simulink model "CardioVascularSystemWithEcmo"  (R2021b)
settings: Solver=daessc  StartTime=0.0  StopTime=Tend  MaxStep=0.6  RelTol=1e-3  AbsTol=1e-3
undefined symbols (not defined in the file): EsL, EsR, PipL, PipR, R1, R2, R3, R4, R5, R6, R7, R8, RL, RPM_Setting, RR, SetHartRate, tc, ts, WaitTime
libraries: fl_lib x66, nesl_utility x24, ee_lib x4, SignalEditorBlockLib x1
settings Model: Creator=mnord  LastModifiedBy=mnord
settings SolverCC: ZeroCrossAlgorithm=Adaptive  AlgebraicLoopSolver=TrustRegion
settings DebuggingCC: MaxConsecutiveZCsMsg=warning  IgnoredZcDiagnostic=none  SymbolicDimsDataTypeCodeGenerationDiagnostic=none  SFMachineParentedDataDiag=warning
settings SFSimCC: CustomCodeUndefinedFunction=UseInterfaceOnly
settings SimscapeCC: SimscapeLogType=all  SimscapeLogSimulationStatistics=on  SimscapeLogDataHistory=10000

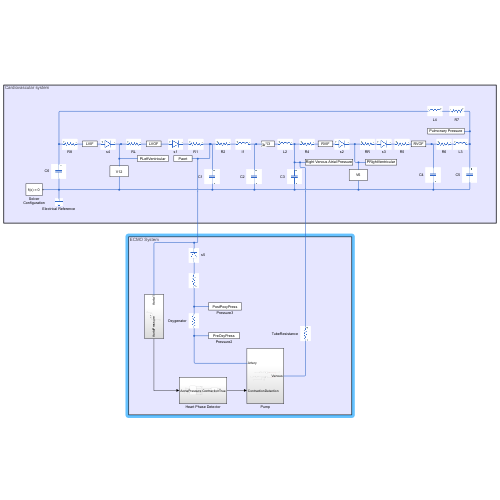
[thumbnail: Simulink's stored preview of the top-level diagram]
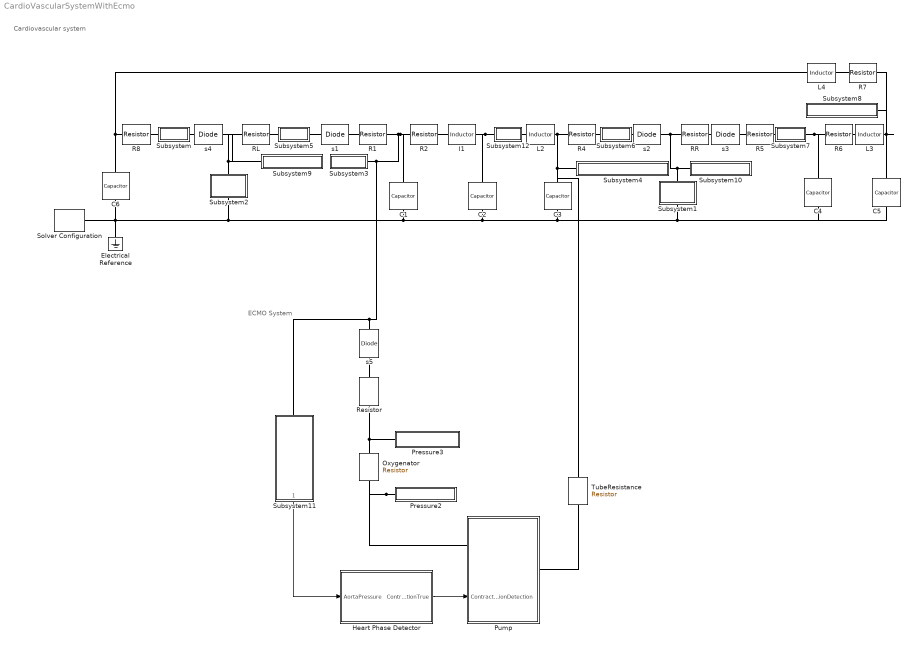
== system CardioVascularSystemWithEcmo ==
  note: Cardiovascular system
  note: ECMO System
  C1 : fl_lib/Electrical/Electrical Elements/Capacitor  c=C1 F  r=capSerRes Ohm  g=0 1/Ohm  i_specify=off  i_priority=None  i=0 A  i_nominal_specify=off  i_nominal_unit=A  i_nominal_value=1  v_specify=off  v_priority=High  v=X10 V  v_nominal_specify=off  v_nominal_unit=V  v_nominal_value=1  vc_specify=on  vc_priority=High  vc=X10 V  vc_nominal_specify=off  vc_nominal_unit=V  vc_nominal_value=1
  C2 : fl_lib/Electrical/Electrical Elements/Capacitor  c=C2 F  r=capSerRes Ohm  g=0 1/Ohm  i_specify=off  i_priority=None  i=0 A  i_nominal_specify=off  i_nominal_unit=A  i_nominal_value=1  v_specify=off  v_priority=High  v=X30 V  v_nominal_specify=off  v_nominal_unit=V  v_nominal_value=1  vc_specify=on  vc_priority=High  vc=X30 V  vc_nominal_specify=off  vc_nominal_unit=V  vc_nominal_value=1
  C3 : fl_lib/Electrical/Electrical Elements/Capacitor  c=C3 F  r=capSerRes Ohm  g=0 1/Ohm  i_specify=off  i_priority=None  i=0 A  i_nominal_specify=off  i_nominal_unit=A  i_nominal_value=1  v_specify=off  v_priority=High  v=X50 V  v_nominal_specify=off  v_nominal_unit=V  v_nominal_value=1  vc_specify=on  vc_priority=High  vc=X50 V  vc_nominal_specify=off  vc_nominal_unit=V  vc_nominal_value=1
  C4 : fl_lib/Electrical/Electrical Elements/Capacitor  c=C4 F  r=capSerRes Ohm  g=0 1/Ohm  i_specify=off  i_priority=None  i=0 A  i_nominal_specify=off  i_nominal_unit=A  i_nominal_value=1  v_specify=off  v_priority=High  v=X70 V  v_nominal_specify=off  v_nominal_unit=V  v_nominal_value=1  vc_specify=on  vc_priority=High  vc=X70 V  vc_nominal_specify=off  vc_nominal_unit=V  vc_nominal_value=1
  C5 : fl_lib/Electrical/Electrical Elements/Capacitor  c=C5 F  r=capSerRes Ohm  g=0 1/Ohm  i_specify=off  i_priority=None  i=0 A  i_nominal_specify=off  i_nominal_unit=A  i_nominal_value=1  v_specify=off  v_priority=High  v=X90 V  v_nominal_specify=off  v_nominal_unit=V  v_nominal_value=1  vc_specify=on  vc_priority=High  vc=X90 V  vc_nominal_specify=off  vc_nominal_unit=V  vc_nominal_value=1
  C6 : fl_lib/Electrical/Electrical Elements/Capacitor  c=C6 F  r=capSerRes Ohm  g=0 1/Ohm  i_specify=off  i_priority=None  i=0 A  i_nominal_specify=off  i_nominal_unit=A  i_nominal_value=1  v_specify=off  v_priority=High  v=X110 V  v_nominal_specify=off  v_nominal_unit=V  v_nominal_value=1  vc_specify=on  vc_priority=High  vc=X110 V  vc_nominal_specify=off  vc_nominal_unit=V  vc_nominal_value=1
  Electrical Reference : fl_lib/Electrical/Electrical Elements/Electrical Reference
  Heart Phase Detector : Subsystem
  I1 : ee_lib/Passive/Inductor  l=L1 H  L_tol=20  enable_L_tol=0  tol_distribution=1  nSigma=4  r=0 Ohm  g=1e-9 1/Ohm  enable_operating_limits=0  operating_limit_action=2  max_working_current=1 A  power_rating=1 W  enable_faults=0  fault_action=1  lambdaPercent=50  k_faulted=0.9999  turnsShort=0  openCct=0  groundShort=0  groundShortG=0 1/Ohm  tau_fault=1e-3 s  enable_temporal_fault=0  t_fault=1 s  enable_behavioral_fault=0  max_permissible_voltage=100 V  n_fail_on_voltage=1  max_permissible_current=1 A  t_fail_on_current=1 s  i_L_specify=on  i_L_priority=High  i_L=X20 A  i_L_nominal_specify=off  i_L_nominal_unit=A  i_L_nominal_value=1
  L2 : ee_lib/Passive/Inductor  l=L2 H  L_tol=20  enable_L_tol=0  tol_distribution=1  nSigma=4  r=0 Ohm  g=1e-9 1/Ohm  enable_operating_limits=0  operating_limit_action=2  max_working_current=1 A  power_rating=1 W  enable_faults=0  fault_action=1  lambdaPercent=50  k_faulted=0.9999  turnsShort=0  openCct=0  groundShort=0  groundShortG=0 1/Ohm  tau_fault=1e-3 s  enable_temporal_fault=0  t_fault=1 s  enable_behavioral_fault=0  max_permissible_voltage=100 V  n_fail_on_voltage=1  max_permissible_current=1 A  t_fail_on_current=1 s  i_L_specify=on  i_L_priority=High  i_L=X40 A  i_L_nominal_specify=off  i_L_nominal_unit=A  i_L_nominal_value=1
  L3 : ee_lib/Passive/Inductor  l=L3 H  L_tol=20  enable_L_tol=0  tol_distribution=1  nSigma=4  r=0 Ohm  g=1e-9 1/Ohm  enable_operating_limits=0  operating_limit_action=2  max_working_current=1 A  power_rating=1 W  enable_faults=0  fault_action=1  lambdaPercent=50  k_faulted=0.9999  turnsShort=0  openCct=0  groundShort=0  groundShortG=0 1/Ohm  tau_fault=1e-3 s  enable_temporal_fault=0  t_fault=1 s  enable_behavioral_fault=0  max_permissible_voltage=100 V  n_fail_on_voltage=1  max_permissible_current=1 A  t_fail_on_current=1 s  i_L_specify=on  i_L_priority=High  i_L=X80 A  i_L_nominal_specify=off  i_L_nominal_unit=A  i_L_nominal_value=1
  L4 : ee_lib/Passive/Inductor  l=L4 H  L_tol=20  enable_L_tol=0  tol_distribution=1  nSigma=4  r=0 Ohm  g=1e-9 1/Ohm  enable_operating_limits=0  operating_limit_action=2  max_working_current=1 A  power_rating=1 W  enable_faults=0  fault_action=1  lambdaPercent=50  k_faulted=0.9999  turnsShort=0  openCct=0  groundShort=0  groundShortG=0 1/Ohm  tau_fault=1e-3 s  enable_temporal_fault=0  t_fault=1 s  enable_behavioral_fault=0  max_permissible_voltage=100 V  n_fail_on_voltage=1  max_permissible_current=1 A  t_fail_on_current=1 s  i_L_specify=on  i_L_priority=High  i_L=X100 A  i_L_nominal_specify=off  i_L_nominal_unit=A  i_L_nominal_value=1
  Oxygenator : fl_lib/Electrical/Electrical Elements/Resistor  R=1/1.13 Ohm  i_specify=off  i_priority=None  i=0 A  i_nominal_specify=off  i_nominal_unit=A  i_nominal_value=1  v_specify=off  v_priority=None  v=0 V  v_nominal_specify=off  v_nominal_unit=V  v_nominal_value=1
  Pressure2 : Subsystem
      mask Display: disp('PreOxyPress')
  Pressure3 : Subsystem
      mask Display: disp('PostPoxyPress')
  Pump : Subsystem
      settings: PortSchema="{\"entries\":[{\"content\":{\"sides\":[{\"content\":{\"connectorIds\":[\"LConn1\"]},\"type\":\"ConnectorPlacement.EquallySpacedRectSide\",\"uuid\":\"62db16dc-542a-4803-9c2c-9a470fc91885\"},{\"content\":{\"connectorIds\":[\"RConn1\",\"In1\"],\"side\":\"RIGHT\"},\"type\":\"ConnectorPlacement.EquallySpacedRectSide\",\"uuid\":\"05a4665e-1cd6-4c93-95ba-f78495d840a1\"},{\"content\":{\"connectorIds\":[],\"side\":\"TOP\"},\"type\":\"ConnectorPlacement.EquallySpacedRectSide\",\"uuid\":\"174192fa-e994-4b45-8a1f-dd44ebe2b866\"},{\"content\":{\"connectorIds\":[],\"side\":\"BOTTOM\"},\"type\":\"ConnectorPlacement.EquallySpacedRectSide\",\"uuid\":\"194a326f-2a13-4189-b0b8-d4f935dc1fe6\"}]},\"type\":\"ConnectorPlacement.EquallySpacedConnector\",\"uuid\":\"9d7b36c7-1763-48ea-a53e-009c812e3b66\"}],\"packageUris\":[\"http://schema.mathworks.com/mf0/Connector/R2020b\"],\"version\":\"1.0\"}"
  R1 : fl_lib/Electrical/Electrical Elements/Resistor  R=R1 Ohm  i_specify=off  i_priority=None  i=0 A  i_nominal_specify=off  i_nominal_unit=A  i_nominal_value=1  v_specify=off  v_priority=None  v=0 V  v_nominal_specify=off  v_nominal_unit=V  v_nominal_value=1
  R2 : fl_lib/Electrical/Electrical Elements/Resistor  R=R2 Ohm  i_specify=off  i_priority=None  i=0 A  i_nominal_specify=off  i_nominal_unit=A  i_nominal_value=1  v_specify=off  v_priority=None  v=0 V  v_nominal_specify=off  v_nominal_unit=V  v_nominal_value=1
  R4 : fl_lib/Electrical/Electrical Elements/Resistor  R=R4 Ohm  i_specify=off  i_priority=None  i=0 A  i_nominal_specify=off  i_nominal_unit=A  i_nominal_value=1  v_specify=off  v_priority=None  v=0 V  v_nominal_specify=off  v_nominal_unit=V  v_nominal_value=1
  R5 : fl_lib/Electrical/Electrical Elements/Resistor  R=R5 Ohm  i_specify=off  i_priority=None  i=0 A  i_nominal_specify=off  i_nominal_unit=A  i_nominal_value=1  v_specify=off  v_priority=None  v=0 V  v_nominal_specify=off  v_nominal_unit=V  v_nominal_value=1
  R6 : fl_lib/Electrical/Electrical Elements/Resistor  R=R6 Ohm  i_specify=off  i_priority=None  i=0 A  i_nominal_specify=off  i_nominal_unit=A  i_nominal_value=1  v_specify=off  v_priority=None  v=0 V  v_nominal_specify=off  v_nominal_unit=V  v_nominal_value=1
  R7 : fl_lib/Electrical/Electrical Elements/Resistor  R=R7 Ohm  i_specify=off  i_priority=None  i=0 A  i_nominal_specify=off  i_nominal_unit=A  i_nominal_value=1  v_specify=off  v_priority=None  v=0 V  v_nominal_specify=off  v_nominal_unit=V  v_nominal_value=1
  R8 : fl_lib/Electrical/Electrical Elements/Resistor  R=R8 Ohm  i_specify=off  i_priority=None  i=0 A  i_nominal_specify=off  i_nominal_unit=A  i_nominal_value=1  v_specify=off  v_priority=None  v=0 V  v_nominal_specify=off  v_nominal_unit=V  v_nominal_value=1
  RL : fl_lib/Electrical/Electrical Elements/Resistor  R=RL Ohm  i_specify=off  i_priority=None  i=0 A  i_nominal_specify=off  i_nominal_unit=A  i_nominal_value=1  v_specify=off  v_priority=None  v=0 V  v_nominal_specify=off  v_nominal_unit=V  v_nominal_value=1
  RR : fl_lib/Electrical/Electrical Elements/Resistor  R=RR Ohm  i_specify=off  i_priority=None  i=0 A  i_nominal_specify=off  i_nominal_unit=A  i_nominal_value=1  v_specify=off  v_priority=None  v=0 V  v_nominal_specify=off  v_nominal_unit=V  v_nominal_value=1
  Resistor : fl_lib/Electrical/Electrical Elements/Resistor  R=1/1.6 Ohm  i_specify=off  i_priority=None  i=0 A  i_nominal_specify=off  i_nominal_unit=A  i_nominal_value=1  v_specify=off  v_priority=None  v=0 V  v_nominal_specify=off  v_nominal_unit=V  v_nominal_value=1
  Solver Configuration : nesl_utility/Solver Configuration  PhysicalDomain=network_engine_domain  SubClassName=solver  LeftPortType=input  RightPortType=generic  Tones=[]  Harmonics=[]  SimulateNoise=off  Profile=off  UseLocalSampling=off  EnableSwitchedLinearOptims=on  FrequencyDomain=off  UseCCode=off  RelTol=0.001  AbsTol=1e-06  MinStep=1e-09  ToWorkspace=off  RevertToSquareIcSolve=off  NumHomotopyIterations=100  PhasorMode=off  PhasorModeNumHarmonics=1  DoDC=off  ResidualTolerance=1e-09  UseLocalSolver=off  LocalSolverChoice=NE_BACKWARD_EULER_ADVANCER  LocalSolverSampleTime=0.001  DoFixedCost=off  MaxNonlinIter=3  MaxModeIter=2  ComputeImpulses=off  ImpulseIterations=2  LinearAlgebra=auto  EquationFormulation=NE_TIME_EF  DelaysMemoryBudget=1024  AutomaticFiltering=on  FilteringTimeConstant=0.001  PartitionStorageMethod=AS_NEEDED  PartitionMemoryBudget=1024  PartitionMethod=ROBUST
      settings: SourceProductBaseCode=PW,SS
  Subsystem : Subsystem
      mask Display: disp('LVIF')
  Subsystem1 : Subsystem
      mask Display: disp('V6')
  Subsystem10 : Subsystem
      mask Display: disp('PRightVentricular')
  Subsystem11 : Subsystem
      settings: PortSchema="{\"entries\":[{\"content\":{\"sides\":[{\"content\":{\"connectorIds\":[]},\"type\":\"ConnectorPlacement.EquallySpacedRectSide\",\"uuid\":\"f9ffc3b3-0f3f-4df5-be7e-a65199d8fb18\"},{\"content\":{\"connectorIds\":[],\"side\":\"RIGHT\"},\"type\":\"ConnectorPlacement.EquallySpacedRectSide\",\"uuid\":\"6b3c46a3-b656-482e-b0a9-93777308e083\"},{\"content\":{\"connectorIds\":[\"LConn1\"],\"side\":\"TOP\"},\"type\":\"ConnectorPlacement.EquallySpacedRectSide\",\"uuid\":\"e2309b6a-a528-4e82-8df5-2fdb2444f40a\"},{\"content\":{\"connectorIds\":[\"Out1\"],\"side\":\"BOTTOM\"},\"type\":\"ConnectorPlacement.EquallySpacedRectSide\",\"uuid\":\"7e89f23f-224f-485d-9e96-fb39bd2403a7\"}]},\"type\":\"ConnectorPlacement.EquallySpacedConnector\",\"uuid\":\"798f20cf-0f77-4082-bc02-f5f2bf5391c0\"}],\"packageUris\":[\"http://schema.mathworks.com/mf0/Connector/R2020b\"],\"version\":\"1.0\"}"
  Subsystem12 : Subsystem  Variant=on  VariantControlMode=label  VariantControl=Choice  LabelModeActiveChoice=R3_Fix
      mask Display: disp('R3')
  Subsystem2 : Subsystem
      mask Display: disp('V12')
  Subsystem3 : Subsystem
      mask Display: disp('Paort')
  Subsystem4 : Subsystem
      mask Display: disp('Right Venous Atrial Pressure')
  Subsystem5 : Subsystem
      mask Display: disp('LVOF')
  Subsystem6 : Subsystem
      mask Display: disp('RVIF')
  Subsystem7 : Subsystem
      mask Display: disp('RVOF')
  Subsystem8 : Subsystem
      mask Display: disp('Pulmonary Pressure')
  Subsystem9 : Subsystem
      mask Display: disp('PLeftVentricular')
  TubeResistance : fl_lib/Electrical/Electrical Elements/Resistor  R=1 Ohm  i_specify=off  i_priority=None  i=60 A  i_nominal_specify=off  i_nominal_unit=A  i_nominal_value=1  v_specify=off  v_priority=None  v=0 V  v_nominal_specify=off  v_nominal_unit=V  v_nominal_value=1
  s{1..4} (4 alike) : fl_lib/Electrical/Electrical Elements/Diode  Vf=FwVolt V  Ron=onRes Ohm  Goff=1e-8 1/Ohm  i_specify=off  i_priority=None  i=0 A  i_nominal_specify=off  i_nominal_unit=A  i_nominal_value=1  v_specify=off  v_priority=None  v=0 V  v_nominal_specify=off  v_nominal_unit=V  v_nominal_value=1
  s5 : fl_lib/Electrical/Electrical Elements/Diode  Vf=FwVolt V  Ron=0.54*0.1 Ohm  Goff=1e-8 1/Ohm  i_specify=off  i_priority=None  i=0 A  i_nominal_specify=off  i_nominal_unit=A  i_nominal_value=1  v_specify=off  v_priority=None  v=0 V  v_nominal_specify=off  v_nominal_unit=V  v_nominal_value=1
  wires:
  Subsystem11/1(AortaPressure) -> Heart Phase Detector/1(AortaPressure)
  Heart Phase Detector/1(ContractionTrue) -> Pump/1(ContractionDetection)
  connections:
  R2/RConn1 -- I1/LConn1
  s1/LConn1 -- Subsystem5/RConn1
  s2/LConn1 -- Subsystem6/RConn1
  R5/RConn1 -- Subsystem7/LConn1
  s4/LConn1 -- Subsystem/RConn1
  R6/LConn1 -- C4/LConn1 -- Subsystem7/RConn1
  Subsystem12/RConn1 -- L2/LConn1
  Subsystem5/LConn1 -- RL/RConn1
  L3/RConn1 -- Subsystem8/LConn1 -- R7/LConn1 -- C5/LConn1
  Subsystem6/LConn1 -- R4/RConn1
  C6/LConn1 -- R8/LConn1 -- L4/RConn1
  s1/RConn1 -- R1/LConn1
  s3/RConn1 -- R5/LConn1
  L3/LConn1 -- R6/RConn1
  R7/RConn1 -- L4/LConn1
  R8/RConn1 -- Subsystem/LConn1
  Subsystem10/LConn1 -- Subsystem1/LConn1 -- RR/LConn1 -- s2/RConn1
  s4/RConn1 -- RL/LConn1 -- Subsystem9/LConn1 -- Subsystem2/LConn1
  s3/LConn1 -- RR/RConn1
  C6/RConn1 -- Electrical Reference/LConn1 -- C5/RConn1 -- C4/RConn1 -- Subsystem1/RConn1 -- C3/RConn1 -- C2/RConn1 -- C1/RConn1 -- Subsystem2/RConn1 -- Solver Configuration/RConn1
  I1/RConn1 -- C2/LConn1 -- Subsystem12/LConn1
  Pressure2/RConn1 -- Pump/RConn1 -- Oxygenator/LConn1
  R4/LConn1 -- TubeResistance/LConn1 -- Subsystem4/LConn1 -- C3/LConn1 -- L2/RConn1
  Resistor/RConn1 -- s5/LConn1
  Oxygenator/RConn1 -- Resistor/LConn1 -- Pressure3/RConn1
  Pump/LConn1 -- TubeResistance/RConn1
  C1/LConn1 -- R1/RConn1 -- Subsystem11/LConn1 -- s5/RConn1 -- Subsystem3/LConn1 -- R2/LConn1

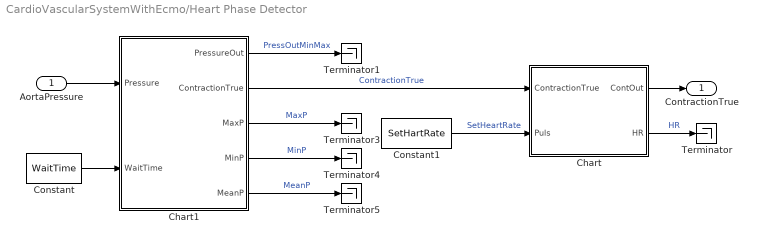
== system CardioVascularSystemWithEcmo/Heart Phase Detector ==
  AortaPressure : Inport
  Chart : Stateflow chart  TreatAsAtomicUnit=on
  Chart1 : Stateflow chart  TreatAsAtomicUnit=on
  Constant : Constant  Value=WaitTime
  Constant1 : Constant  Value=SetHartRate
  Terminator{,1,3..5} (5 alike) : Terminator
  ContractionTrue : Outport
  wires:
  AortaPressure/1 -> Chart1/1(Pressure)
  Chart1/1(PressureOut) -> Terminator1/1  "PressOutMinMax"
  Chart1/2(ContractionTrue) -> Chart/1(ContractionTrue)  "ContractionTrue"
  Chart1/4(MinP) -> Terminator4/1  "MinP"
  Chart1/3(MaxP) -> Terminator3/1  "MaxP"
  Chart1/5(MeanP) -> Terminator5/1  "MeanP"
  Constant/1 -> Chart1/2(WaitTime)
  Chart/1(ContOut) -> ContractionTrue/1
  Chart/2(HR) -> Terminator/1  "HR"
  Constant1/1 -> Chart/2(Puls)  "SetHeartRate"

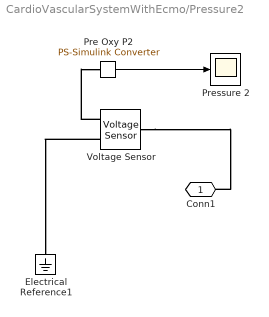
== system CardioVascularSystemWithEcmo/Pressure2 ==
  Electrical Reference1 : fl_lib/Electrical/Electrical Elements/Electrical Reference
  Pre Oxy P2 : nesl_utility/PS-Simulink Converter  PhysicalDomain=network_engine_domain  SubClassName=ps_output  LeftPortType=input  RightPortType=output  PseudoPeriodic=off  Frequencies=[]  Unit=inherit  AffineConversion=off
      settings: SourceProductBaseCode=PW,SS
  Pressure 2 : Scope
  Voltage Sensor : fl_lib/Electrical/Electrical Sensors/Voltage Sensor
  Conn1 : PMIOPort  Side=Right
  wires:
  Pre Oxy P2/1 -> Pressure 2/1
  connections:
  Voltage Sensor/RConn1 -- Pre Oxy P2/LConn1
  Voltage Sensor/LConn1 -- Conn1/RConn1
  Voltage Sensor/RConn2 -- Electrical Reference1/LConn1

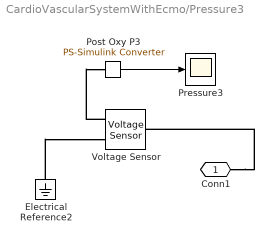
== system CardioVascularSystemWithEcmo/Pressure3 ==
  Electrical Reference2 : fl_lib/Electrical/Electrical Elements/Electrical Reference
  Post Oxy P3 : nesl_utility/PS-Simulink Converter  PhysicalDomain=network_engine_domain  SubClassName=ps_output  LeftPortType=input  RightPortType=output  PseudoPeriodic=off  Frequencies=[]  Unit=inherit  AffineConversion=off
      settings: SourceProductBaseCode=PW,SS
  Pressure3 : Scope
  Voltage Sensor : fl_lib/Electrical/Electrical Sensors/Voltage Sensor
  Conn1 : PMIOPort  Side=Right
  wires:
  Post Oxy P3/1 -> Pressure3/1
  connections:
  Voltage Sensor/RConn1 -- Post Oxy P3/LConn1
  Electrical Reference2/LConn1 -- Voltage Sensor/RConn2
  Conn1/RConn1 -- Voltage Sensor/LConn1

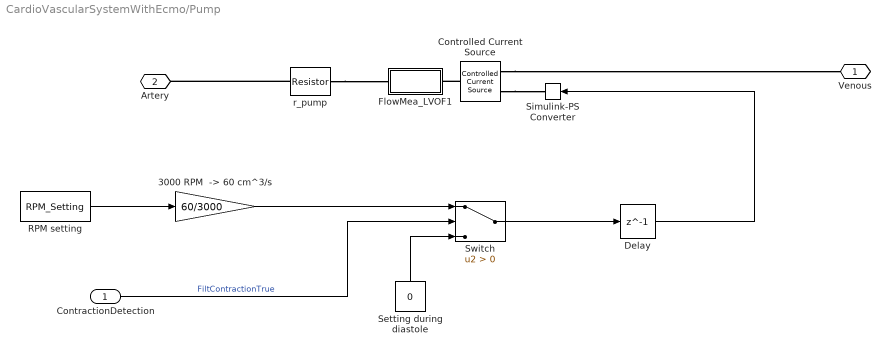
== system CardioVascularSystemWithEcmo/Pump ==
  ContractionDetection : Inport
  "3000 RPM  -> 60 cm^3/s" : Gain  Gain=60/3000
  Controlled Current Source : fl_lib/Electrical/Electrical Sources/Controlled Current Source
  Delay : Delay  DelayLength=1  SampleTime=0.001
  FlowMea_LVOF1 : Subsystem
      mask Display: disp('EcmoFlow')
  RPM setting : Constant  Value=RPM_Setting
  Setting during diastole : Constant  Value=0
  Simulink-PS Converter : nesl_utility/Simulink-PS Converter  PhysicalDomain=network_engine_domain  SubClassName=ps_input  LeftPortType=input  RightPortType=output  PseudoPeriodic=off  Frequencies=[]  NoiseDistribution=none  NoiseParameters=[]  Unit=1  AffineConversion=off  FilteringAndDerivatives=filter  SimscapeFilterOrder=1  InputFilterTimeConstant=0.001  UdotUserProvided=0
      settings: SourceProductBaseCode=PW,SS
  Switch : Switch  Criteria=u2 > Threshold
  r_pump : fl_lib/Electrical/Electrical Elements/Resistor  R=1/1.68 Ohm  i_specify=on  i_priority=None  i=83.3 A  i_nominal_specify=off  i_nominal_unit=A  i_nominal_value=1  v_specify=off  v_priority=None  v=0 V  v_nominal_specify=off  v_nominal_unit=V  v_nominal_value=1
  Venous : PMIOPort  Side=Left
  Artery : PMIOPort  Port=2  Side=Right
  wires:
  Delay/1 -> Simulink-PS Converter/1
  "3000 RPM  -> 60 cm^3/s"/1 -> Switch/1
  ContractionDetection/1 -> Switch/2  "FiltContractionTrue"
  RPM setting/1 -> "3000 RPM  -> 60 cm^3/s"/1
  Switch/1 -> Delay/1
  Setting during diastole/1 -> Switch/3
  connections:
  Controlled Current Source/RConn2 -- Venous/RConn1
  r_pump/LConn1 -- FlowMea_LVOF1/LConn1
  Controlled Current Source/RConn1 -- Simulink-PS Converter/RConn1
  r_pump/RConn1 -- Artery/RConn1
  Controlled Current Source/LConn1 -- FlowMea_LVOF1/RConn1

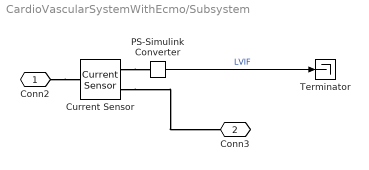
== system CardioVascularSystemWithEcmo/Subsystem ==
  Current Sensor : fl_lib/Electrical/Electrical Sensors/Current Sensor
  PS-Simulink Converter : nesl_utility/PS-Simulink Converter  PhysicalDomain=network_engine_domain  SubClassName=ps_output  LeftPortType=input  RightPortType=output  PseudoPeriodic=off  Frequencies=[]  Unit=inherit  AffineConversion=off
      settings: SourceProductBaseCode=PW,SS
  Terminator : Terminator
  Conn2 : PMIOPort  Side=Left
  Conn3 : PMIOPort  Port=2  Side=Right
  wires:
  PS-Simulink Converter/1 -> Terminator/1  "LVIF"
  connections:
  Conn2/RConn1 -- Current Sensor/LConn1
  Current Sensor/RConn2 -- Conn3/RConn1
  Current Sensor/RConn1 -- PS-Simulink Converter/LConn1

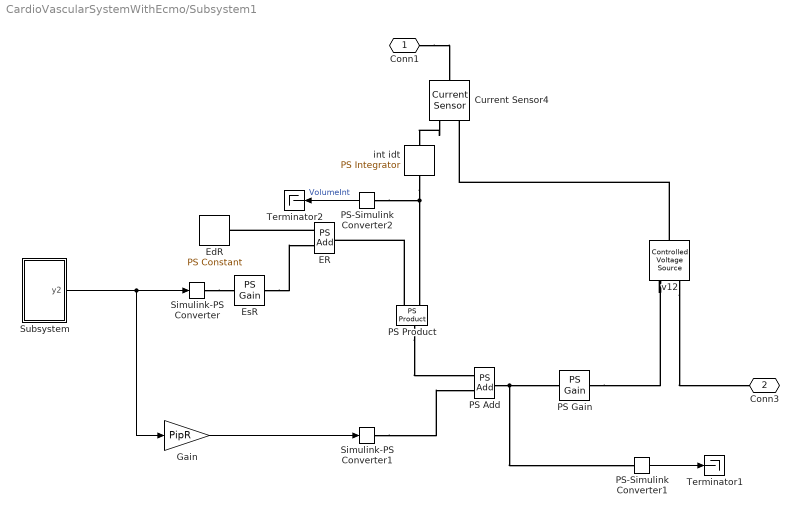
== system CardioVascularSystemWithEcmo/Subsystem1 ==
  Current Sensor4 : fl_lib/Electrical/Electrical Sensors/Current Sensor
  ER : fl_lib/Physical Signals/Functions/PS Add
  EdR : fl_lib/Physical Signals/Sources/PS Constant  constant=EdR
  EsR : fl_lib/Physical Signals/Functions/PS Gain  gain=EsR
  Gain : Gain  Gain=PipR
  PS Add : fl_lib/Physical Signals/Functions/PS Add
  PS Gain : fl_lib/Physical Signals/Functions/PS Gain  gain=1 V/s/A
  PS Product : fl_lib/Physical Signals/Functions/PS Product
  PS-Simulink Converter1 : nesl_utility/PS-Simulink Converter  PhysicalDomain=network_engine_domain  SubClassName=ps_output  LeftPortType=input  RightPortType=output  PseudoPeriodic=off  Frequencies=[]  Unit=inherit  AffineConversion=off
      settings: SourceProductBaseCode=PW,SS
  PS-Simulink Converter2 : nesl_utility/PS-Simulink Converter  PhysicalDomain=network_engine_domain  SubClassName=ps_output  LeftPortType=input  RightPortType=output  PseudoPeriodic=off  Frequencies=[]  Unit=inherit  AffineConversion=off
      settings: SourceProductBaseCode=PW,SS
  Simulink-PS Converter : nesl_utility/Simulink-PS Converter  PhysicalDomain=network_engine_domain  SubClassName=ps_input  LeftPortType=input  RightPortType=output  PseudoPeriodic=off  Frequencies=[]  NoiseDistribution=none  NoiseParameters=[]  Unit=1  AffineConversion=off  FilteringAndDerivatives=provide  SimscapeFilterOrder=1  InputFilterTimeConstant=0.001  UdotUserProvided=0
      settings: SourceProductBaseCode=PW,SS
  Simulink-PS Converter1 : nesl_utility/Simulink-PS Converter  PhysicalDomain=network_engine_domain  SubClassName=ps_input  LeftPortType=input  RightPortType=output  PseudoPeriodic=off  Frequencies=[]  NoiseDistribution=none  NoiseParameters=[]  Unit=A*s  AffineConversion=off  FilteringAndDerivatives=provide  SimscapeFilterOrder=1  InputFilterTimeConstant=0.001  UdotUserProvided=0
      settings: SourceProductBaseCode=PW,SS
  Subsystem : Subsystem
  Terminator1 : Terminator
  Terminator2 : Terminator
  int idt : fl_lib/Physical Signals/Linear Operators/PS Integrator  reset_method=foundation.enum.IntegratorResetSpec.None  initial_condition_spec=foundation.enum.IntegratorICSpec.Internal  x0=X60 A*s
      settings: SourceProductBaseCode=SS
  v12 : fl_lib/Electrical/Electrical Sources/Controlled Voltage Source
  Conn1 : PMIOPort  Side=Left
  Conn3 : PMIOPort  Port=2  Side=Right
  wires:
  PS-Simulink Converter1/1 -> Terminator1/1
  Gain/1 -> Simulink-PS Converter1/1
  PS-Simulink Converter2/1 -> Terminator2/1  "VolumeInt"
  Subsystem/1(y2) -> Gain/1, Simulink-PS Converter/1
  connections:
  PS Add/RConn1 -- PS-Simulink Converter1/LConn1 -- PS Gain/LConn1
  PS-Simulink Converter2/LConn1 -- PS Product/LConn1 -- int idt/RConn1
  PS Product/RConn1 -- PS Add/LConn1
  v12/LConn1 -- Current Sensor4/RConn2
  ER/LConn1 -- EdR/RConn1
  Simulink-PS Converter1/RConn1 -- PS Add/LConn2
  EsR/RConn1 -- ER/LConn2
  PS Product/LConn2 -- ER/RConn1
  v12/RConn2 -- Conn3/RConn1
  Conn1/RConn1 -- Current Sensor4/LConn1
  Current Sensor4/RConn1 -- int idt/LConn1
  Simulink-PS Converter/RConn1 -- EsR/LConn1
  PS Gain/RConn1 -- v12/RConn1

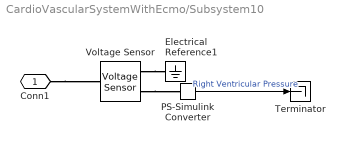
== system CardioVascularSystemWithEcmo/Subsystem10 ==
  Electrical Reference1 : fl_lib/Electrical/Electrical Elements/Electrical Reference
  PS-Simulink Converter : nesl_utility/PS-Simulink Converter  PhysicalDomain=network_engine_domain  SubClassName=ps_output  LeftPortType=input  RightPortType=output  PseudoPeriodic=off  Frequencies=[]  Unit=inherit  AffineConversion=off
      settings: SourceProductBaseCode=PW,SS
  Terminator : Terminator
  Voltage Sensor : fl_lib/Electrical/Electrical Sensors/Voltage Sensor
  Conn1 : PMIOPort  Side=Left
  wires:
  PS-Simulink Converter/1 -> Terminator/1  "Right Ventricular Pressure"
  connections:
  Conn1/RConn1 -- Voltage Sensor/LConn1
  Voltage Sensor/RConn2 -- Electrical Reference1/LConn1
  Voltage Sensor/RConn1 -- PS-Simulink Converter/LConn1

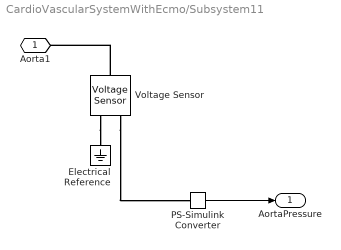
== system CardioVascularSystemWithEcmo/Subsystem11 ==
  Electrical Reference : fl_lib/Electrical/Electrical Elements/Electrical Reference
  PS-Simulink Converter : nesl_utility/PS-Simulink Converter  PhysicalDomain=network_engine_domain  SubClassName=ps_output  LeftPortType=input  RightPortType=output  PseudoPeriodic=off  Frequencies=[]  Unit=inherit  AffineConversion=off
      settings: SourceProductBaseCode=PW,SS
  Voltage Sensor : fl_lib/Electrical/Electrical Sensors/Voltage Sensor
  Aorta1 : PMIOPort  Side=Left
  AortaPressure : Outport
  wires:
  PS-Simulink Converter/1 -> AortaPressure/1
  connections:
  Voltage Sensor/LConn1 -- Aorta1/RConn1
  Voltage Sensor/RConn2 -- Electrical Reference/LConn1
  Voltage Sensor/RConn1 -- PS-Simulink Converter/LConn1

== system CardioVascularSystemWithEcmo/Subsystem12 ==
  Fixed : Subsystem  VariantControl=R3_Fix
  Variable : Subsystem  VariantControl=R3_Variant
  Conn1 : PMIOPort  Side=Left
  Conn2 : PMIOPort  Port=2  Side=Right

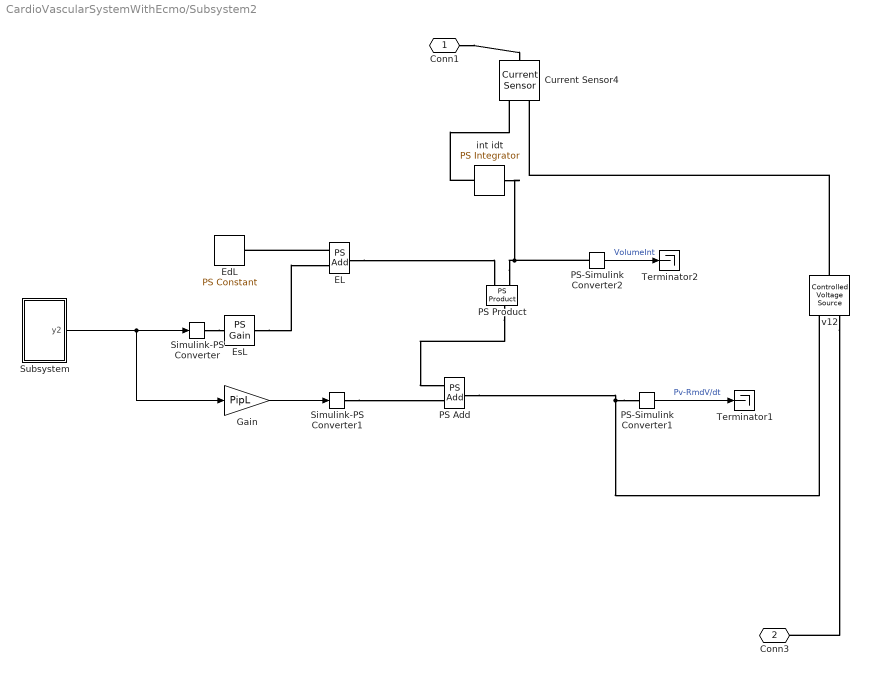
== system CardioVascularSystemWithEcmo/Subsystem2 ==
  Current Sensor4 : fl_lib/Electrical/Electrical Sensors/Current Sensor
  EL : fl_lib/Physical Signals/Functions/PS Add
  EdL : fl_lib/Physical Signals/Sources/PS Constant  constant=EdL V/A/s
  EsL : fl_lib/Physical Signals/Functions/PS Gain  gain=EsL
  Gain : Gain  Gain=PipL
  PS Add : fl_lib/Physical Signals/Functions/PS Add
  PS Product : fl_lib/Physical Signals/Functions/PS Product
  PS-Simulink Converter1 : nesl_utility/PS-Simulink Converter  PhysicalDomain=network_engine_domain  SubClassName=ps_output  LeftPortType=input  RightPortType=output  PseudoPeriodic=off  Frequencies=[]  Unit=inherit  AffineConversion=off
      settings: SourceProductBaseCode=PW,SS
  PS-Simulink Converter2 : nesl_utility/PS-Simulink Converter  PhysicalDomain=network_engine_domain  SubClassName=ps_output  LeftPortType=input  RightPortType=output  PseudoPeriodic=off  Frequencies=[]  Unit=inherit  AffineConversion=off
      settings: SourceProductBaseCode=PW,SS
  Simulink-PS Converter : nesl_utility/Simulink-PS Converter  PhysicalDomain=network_engine_domain  SubClassName=ps_input  LeftPortType=input  RightPortType=output  PseudoPeriodic=off  Frequencies=[]  NoiseDistribution=none  NoiseParameters=[]  Unit=V/A/s  AffineConversion=off  FilteringAndDerivatives=provide  SimscapeFilterOrder=1  InputFilterTimeConstant=0.001  UdotUserProvided=0
      settings: SourceProductBaseCode=PW,SS
  Simulink-PS Converter1 : nesl_utility/Simulink-PS Converter  PhysicalDomain=network_engine_domain  SubClassName=ps_input  LeftPortType=input  RightPortType=output  PseudoPeriodic=off  Frequencies=[]  NoiseDistribution=none  NoiseParameters=[]  Unit=V  AffineConversion=off  FilteringAndDerivatives=provide  SimscapeFilterOrder=1  InputFilterTimeConstant=0.001  UdotUserProvided=0
      settings: SourceProductBaseCode=PW,SS
  Subsystem : Subsystem
  Terminator1 : Terminator
  Terminator2 : Terminator
  int idt : fl_lib/Physical Signals/Linear Operators/PS Integrator  reset_method=foundation.enum.IntegratorResetSpec.None  initial_condition_spec=foundation.enum.IntegratorICSpec.Internal  x0=X120 A*s
      settings: SourceProductBaseCode=SS
  v12 : fl_lib/Electrical/Electrical Sources/Controlled Voltage Source
  Conn1 : PMIOPort  Side=Left
  Conn3 : PMIOPort  Port=2  Side=Right
  wires:
  Gain/1 -> Simulink-PS Converter1/1
  Subsystem/1(y2) -> Gain/1, Simulink-PS Converter/1
  PS-Simulink Converter1/1 -> Terminator1/1  "Pv-RmdV/dt"
  PS-Simulink Converter2/1 -> Terminator2/1  "VolumeInt"
  connections:
  PS Product/LConn1 -- int idt/RConn1 -- PS-Simulink Converter2/LConn1
  EL/LConn1 -- EdL/RConn1
  PS Product/RConn1 -- PS Add/LConn1
  EsL/RConn1 -- EL/LConn2
  Simulink-PS Converter1/RConn1 -- PS Add/LConn2
  Simulink-PS Converter/RConn1 -- EsL/LConn1
  v12/RConn2 -- Conn3/RConn1
  int idt/LConn1 -- Current Sensor4/RConn1
  Conn1/RConn1 -- Current Sensor4/LConn1
  EL/RConn1 -- PS Product/LConn2
  PS-Simulink Converter1/LConn1 -- PS Add/RConn1 -- v12/RConn1
  v12/LConn1 -- Current Sensor4/RConn2

== system CardioVascularSystemWithEcmo/Subsystem3 ==
  Electrical Reference1 : fl_lib/Electrical/Electrical Elements/Electrical Reference
  PS-Simulink Converter : nesl_utility/PS-Simulink Converter  PhysicalDomain=network_engine_domain  SubClassName=ps_output  LeftPortType=input  RightPortType=output  PseudoPeriodic=off  Frequencies=[]  Unit=inherit  AffineConversion=off
      settings: SourceProductBaseCode=PW,SS
  Terminator : Terminator
  Voltage Sensor : fl_lib/Electrical/Electrical Sensors/Voltage Sensor
  Conn1 : PMIOPort  Side=Left
  wires:
  PS-Simulink Converter/1 -> Terminator/1  "Aortic Pressure"
  connections:
  Voltage Sensor/RConn1 -- PS-Simulink Converter/LConn1
  Voltage Sensor/RConn2 -- Electrical Reference1/LConn1
  Conn1/RConn1 -- Voltage Sensor/LConn1

== system CardioVascularSystemWithEcmo/Subsystem4 ==
  Electrical Reference1 : fl_lib/Electrical/Electrical Elements/Electrical Reference
  PS-Simulink Converter : nesl_utility/PS-Simulink Converter  PhysicalDomain=network_engine_domain  SubClassName=ps_output  LeftPortType=input  RightPortType=output  PseudoPeriodic=off  Frequencies=[]  Unit=inherit  AffineConversion=off
      settings: SourceProductBaseCode=PW,SS
  Terminator : Terminator
  Voltage Sensor : fl_lib/Electrical/Electrical Sensors/Voltage Sensor
  Conn1 : PMIOPort  Side=Left
  wires:
  PS-Simulink Converter/1 -> Terminator/1  "Right Venous Atrial Pressure"
  connections:
  Conn1/RConn1 -- Voltage Sensor/LConn1
  Voltage Sensor/RConn2 -- Electrical Reference1/LConn1
  Voltage Sensor/RConn1 -- PS-Simulink Converter/LConn1

== system CardioVascularSystemWithEcmo/Subsystem5 ==
  Current Sensor : fl_lib/Electrical/Electrical Sensors/Current Sensor
  PS-Simulink Converter : nesl_utility/PS-Simulink Converter  PhysicalDomain=network_engine_domain  SubClassName=ps_output  LeftPortType=input  RightPortType=output  PseudoPeriodic=off  Frequencies=[]  Unit=inherit  AffineConversion=off
      settings: SourceProductBaseCode=PW,SS
  Terminator : Terminator
  Conn2 : PMIOPort  Side=Left
  Conn3 : PMIOPort  Port=2  Side=Right
  wires:
  PS-Simulink Converter/1 -> Terminator/1  "LVOF"
  connections:
  Conn2/RConn1 -- Current Sensor/LConn1
  Current Sensor/RConn2 -- Conn3/RConn1
  Current Sensor/RConn1 -- PS-Simulink Converter/LConn1

== system CardioVascularSystemWithEcmo/Subsystem6 ==
  Current Sensor : fl_lib/Electrical/Electrical Sensors/Current Sensor
  PS-Simulink Converter : nesl_utility/PS-Simulink Converter  PhysicalDomain=network_engine_domain  SubClassName=ps_output  LeftPortType=input  RightPortType=output  PseudoPeriodic=off  Frequencies=[]  Unit=inherit  AffineConversion=off
      settings: SourceProductBaseCode=PW,SS
  Terminator : Terminator
  Conn2 : PMIOPort  Side=Left
  Conn3 : PMIOPort  Port=2  Side=Right
  wires:
  PS-Simulink Converter/1 -> Terminator/1  "RVIF"
  connections:
  Current Sensor/RConn1 -- PS-Simulink Converter/LConn1
  Current Sensor/RConn2 -- Conn3/RConn1
  Conn2/RConn1 -- Current Sensor/LConn1

== system CardioVascularSystemWithEcmo/Subsystem7 ==
  Current Sensor : fl_lib/Electrical/Electrical Sensors/Current Sensor
  PS-Simulink Converter : nesl_utility/PS-Simulink Converter  PhysicalDomain=network_engine_domain  SubClassName=ps_output  LeftPortType=input  RightPortType=output  PseudoPeriodic=off  Frequencies=[]  Unit=inherit  AffineConversion=off
      settings: SourceProductBaseCode=PW,SS
  Terminator : Terminator
  Conn2 : PMIOPort  Side=Left
  Conn3 : PMIOPort  Port=2  Side=Right
  wires:
  PS-Simulink Converter/1 -> Terminator/1  "RVOF"
  connections:
  Conn2/RConn1 -- Current Sensor/LConn1
  Current Sensor/RConn2 -- Conn3/RConn1
  Current Sensor/RConn1 -- PS-Simulink Converter/LConn1

== system CardioVascularSystemWithEcmo/Subsystem8 ==
  Electrical Reference1 : fl_lib/Electrical/Electrical Elements/Electrical Reference
  PS-Simulink Converter : nesl_utility/PS-Simulink Converter  PhysicalDomain=network_engine_domain  SubClassName=ps_output  LeftPortType=input  RightPortType=output  PseudoPeriodic=off  Frequencies=[]  Unit=inherit  AffineConversion=off
      settings: SourceProductBaseCode=PW,SS
  Terminator : Terminator
  Voltage Sensor : fl_lib/Electrical/Electrical Sensors/Voltage Sensor
  Conn1 : PMIOPort  Side=Left
  wires:
  PS-Simulink Converter/1 -> Terminator/1  "Pulmonary Pressure"
  connections:
  Conn1/RConn1 -- Voltage Sensor/LConn1
  Voltage Sensor/RConn2 -- Electrical Reference1/LConn1
  Voltage Sensor/RConn1 -- PS-Simulink Converter/LConn1

== system CardioVascularSystemWithEcmo/Subsystem9 ==
  Electrical Reference1 : fl_lib/Electrical/Electrical Elements/Electrical Reference
  PS-Simulink Converter : nesl_utility/PS-Simulink Converter  PhysicalDomain=network_engine_domain  SubClassName=ps_output  LeftPortType=input  RightPortType=output  PseudoPeriodic=off  Frequencies=[]  Unit=inherit  AffineConversion=off
      settings: SourceProductBaseCode=PW,SS
  Terminator : Terminator
  Voltage Sensor : fl_lib/Electrical/Electrical Sensors/Voltage Sensor
  Conn1 : PMIOPort  Side=Left
  wires:
  PS-Simulink Converter/1 -> Terminator/1  "Left Ventricular Pressure"
  connections:
  Conn1/RConn1 -- Voltage Sensor/LConn1
  Voltage Sensor/RConn2 -- Electrical Reference1/LConn1
  Voltage Sensor/RConn1 -- PS-Simulink Converter/LConn1

== system CardioVascularSystemWithEcmo/Pump/FlowMea_LVOF1 ==
  Current Sensor3 : fl_lib/Electrical/Electrical Sensors/Current Sensor
  ECMOflow : Scope
  PS-Simulink Converter6 : nesl_utility/PS-Simulink Converter  PhysicalDomain=network_engine_domain  SubClassName=ps_output  LeftPortType=input  RightPortType=output  PseudoPeriodic=off  Frequencies=[]  Unit=inherit  AffineConversion=on
      settings: SourceProductBaseCode=PW,SS
  Out : PMIOPort  Side=Left
  In : PMIOPort  Port=2  Side=Right
  wires:
  PS-Simulink Converter6/1 -> ECMOflow/1  "ECMOflow"
  connections:
  Current Sensor3/RConn1 -- PS-Simulink Converter6/LConn1
  Current Sensor3/LConn1 -- In/RConn1
  Current Sensor3/RConn2 -- Out/RConn1

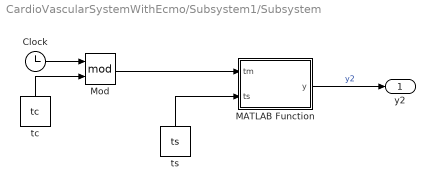
== system CardioVascularSystemWithEcmo/Subsystem1/Subsystem ==
  Clock : Clock
  MATLAB Function : MATLAB Function  TreatAsAtomicUnit=on
  Mod : Math  Operator=mod  SaturateOnIntegerOverflow=on
  tc : Constant  Value=tc
  ts : Constant  Value=ts
  y2 : Outport
  wires:
  Clock/1 -> Mod/1
  Mod/1 -> MATLAB Function/1(tm)
  MATLAB Function/1(y) -> y2/1  "y2"
  ts/1 -> MATLAB Function/2(ts)
  tc/1 -> Mod/2

== system CardioVascularSystemWithEcmo/Subsystem12/Fixed ==
  R3 : fl_lib/Electrical/Electrical Elements/Resistor  R=R3 Ohm  i_specify=off  i_priority=None  i=0 A  i_nominal_specify=off  i_nominal_unit=A  i_nominal_value=1  v_specify=off  v_priority=None  v=0 V  v_nominal_specify=off  v_nominal_unit=V  v_nominal_value=1
  Conn1 : PMIOPort  Side=Left
  Conn2 : PMIOPort  Port=2  Side=Right
  connections:
  R3/RConn1 -- Conn2/RConn1
  R3/LConn1 -- Conn1/RConn1

== system CardioVascularSystemWithEcmo/Subsystem12/Variable ==
  Signal Editor : SignalEditorBlockLib/Signal Editor  FileName=R3_Values.mat  ActiveScenario=Scenario  ActiveSignal=Signal 1  IsBus=off  OutputBusObjectStr=Bus: BusObject  SampleTime=0  Interpolate=off  ZeroCross=off  OutputAfterFinalValue=Holding final value  Unit=inherit  PreserveSignalName=on
  Simulink-PS Converter : nesl_utility/Simulink-PS Converter  PhysicalDomain=network_engine_domain  SubClassName=ps_input  LeftPortType=input  RightPortType=output  PseudoPeriodic=off  Frequencies=[]  NoiseDistribution=none  NoiseParameters=[]  Unit=1  AffineConversion=off  FilteringAndDerivatives=provide  SimscapeFilterOrder=1  InputFilterTimeConstant=0.001  UdotUserProvided=0
      settings: SourceProductBaseCode=PW,SS
  Variable Resistor : fl_lib/Electrical/Electrical Elements/Variable Resistor  Rmin=0 Ohm  i_specify=off  i_priority=None  i=0 A  i_nominal_specify=off  i_nominal_unit=A  i_nominal_value=1  v_specify=off  v_priority=None  v=0 V  v_nominal_specify=off  v_nominal_unit=V  v_nominal_value=1
  Conn1 : PMIOPort  Side=Left
  Conn2 : PMIOPort  Port=2  Side=Right
  wires:
  Signal Editor/1 -> Simulink-PS Converter/1  "R3_ohm"
  connections:
  Variable Resistor/LConn1 -- Simulink-PS Converter/RConn1
  Variable Resistor/RConn1 -- Conn2/RConn1
  Variable Resistor/LConn2 -- Conn1/RConn1

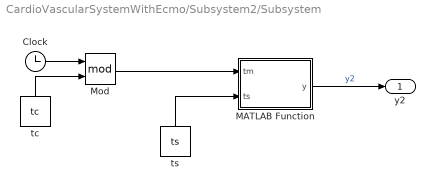
== system CardioVascularSystemWithEcmo/Subsystem2/Subsystem ==
  Clock : Clock
  MATLAB Function : MATLAB Function  TreatAsAtomicUnit=on
  Mod : Math  Operator=mod  SaturateOnIntegerOverflow=on
  tc : Constant  Value=tc
  ts : Constant  Value=ts
  y2 : Outport
  wires:
  Clock/1 -> Mod/1
  Mod/1 -> MATLAB Function/1(tm)
  MATLAB Function/1(y) -> y2/1  "y2"
  ts/1 -> MATLAB Function/2(ts)
  tc/1 -> Mod/2

== matlab function CardioVascularSystemWithEcmo/Subsystem1/Subsystem/MATLAB Function ==
  data: tm input; y output; ts input
function y = fcn(tm, ts)

if(tm< ts)
    y = (1-cos(2*pi*tm/ts)) * 0.5;
else
    y = 0;
end

== matlab function CardioVascularSystemWithEcmo/Subsystem2/Subsystem/MATLAB Function ==
  data: tm input; y output; ts input
function y = fcn(tm, ts)

if(tm< ts)
    y = (1-cos(2*pi*tm/ts)) * 0.5;
else
    y = 0;
end

== stateflow chart CardioVascularSystemWithEcmo/Heart Phase Detector/Chart ==
  state HR_calc [parallel]
    settings: executionOrder=1
    state Init
      OffTime = 0;
      HR = 90;
    state On
      ex:
      %ONtime = elapsed(sec);
      ONtime = max(1/HR*0.2,elapsed(sec));
      HR = 0.5*HR + 0.5*60/( OffTime + ONtime);
      HR = min(220,HR);
      HR = max(50,HR);
      HR = Puls; % Override with set Pulse
    state Off
      du:
      OffTime = elapsed(sec);
    (default) -> Init
    Init -> HR_calc.On
    Off -> HR_calc.On : [ContractionTrue == true]
    HR_calc.On -> Off : [ContractionTrue == false]
  state CalcOutput [parallel]
    settings: executionOrder=2
    state On
      du:
      ContOut = true;
    state HRlessThan140
      du:
      ContOut = false;
    state HRMoreThan150
      % Inhibit true #1
      du:
      ContOut = false;
    state HRmoreThan140lessThan150
      % Inhibit true #1
      en:
      ContOut = false;
    state LastFalse
      ContOut = false;
    state False
      ContOut = false;
    state ThirdInhabitedTrue
      % Inhibit true #2
      ContOut = false;
    (default) -> CalcOutput.On
    HRlessThan140 -> CalcOutput.On [order 1] : [ContractionTrue == true & HR <140]
    HRlessThan140 -> HRMoreThan150 [order 3] : [ContractionTrue== true] % HR >= 150
    CalcOutput.On -> HRlessThan140 : [ContractionTrue==false]
    LastFalse -> CalcOutput.On : [ContractionTrue==true]
    HRlessThan140 -> HRmoreThan140lessThan150 [order 2] : [ContractionTrue == true  & true & HR < 150]
    HRmoreThan140lessThan150 -> LastFalse : [ContractionTrue == false ]
    HRMoreThan150 -> False : [ContractionTrue == false]
    ThirdInhabitedTrue -> LastFalse : [ContractionTrue==false]
    False -> ThirdInhabitedTrue : [ContractionTrue == true]
  data: ContractionTrue input; ContOut output; ONtime local; OffTime local; HR output; Puls input

== stateflow chart CardioVascularSystemWithEcmo/Heart Phase Detector/Chart1 ==
  state Contracton
    du:
    MaxP = max(Pressure,MaxP);
    ContractionTrue = true;
    PressureOut = Pressure;
    MeanP = Pressure/1000+...
    999*MeanP/1000;
    LastP = Pressure;
  state Hold
    du:
    MaxP = max(Pressure,MaxP);
    ContractionTrue = true;
    PressureOut = Pressure;
    MeanP = Pressure/1000+...
    999*MeanP/1000;
    LastP = Pressure;
  state Init
    en:
    MaxP=Pressure;
    MinP = Pressure;
    MeanP = 50;
    LastP = Pressure;
  state NoContraction
    state NoContractionHold
      du:
      MinP = min(Pressure,MinP);
      ContractionTrue = false;
      PressureOut = 0;
      MeanP = Pressure/1000+...
      999*MeanP/1000;
      LastP = Pressure;
    state NoContraction
      du:
      MinP = min(Pressure,MinP);
      ContractionTrue = false;
      PressureOut = 0;
      MeanP = Pressure/1000+...
      999*MeanP/1000;
      LastP = Pressure;
    NoContractionHold -> NoContraction.NoContraction [order 2] : [LastP > Pressure]
    NoContraction.NoContraction -> NoContractionHold : [LastP<Pressure]
  (default) -> Init
  Init -> Contracton
  Contracton -> Hold : [LastP > Pressure]
  Hold -> Contracton [order 2] : [LastP<Pressure]
  Hold -> NoContraction.NoContraction [order 1] : after(WaitTime,sec){MaxP = Pressure;}
  NoContractionHold -> Contracton [order 1] : [after(WaitTime,sec) & Pressure < MeanP]{MinP = Pressure;}
  data: Pressure input; PressureOut output; ContractionTrue output; MaxP output; MinP output; MeanP output; LastP local; WaitTime input
